simulink model "demoProxyRPi"  (R2016a)
settings: Solver=FixedStepAuto  StartTime=0.0  StopTime=inf  FixedStep=1  RelTol=1e-3
undefined symbols (not defined in the file): Green, led0
libraries: embdlinuxlib x3, RPi x2
settings Model: SimulationMode=external  Creator=user  LastModifiedBy=user
settings SolverCC: PositivePriorityOrder=on
settings OptimizationCC: OptimizeModelRefInitCode=on  LifeSpan=1  MaxStackSize=64
settings HardwareCC: ProdBitPerPointer=32  ProdLargestAtomicInteger=Long  ProdLargestAtomicFloat=Double  ProdWordSize=32  ProdHWDeviceType=ARM Compatible->ARM Cortex
settings RTWCC: SystemTargetFile=ert.tlc  HardwareBoard=Raspberry Pi  TemplateMakefile=ert_default_tmf  GenerateReport=on  Toolchain=GNU GCC Raspberry Pi  IncludeHyperlinkInReport=on  LaunchReport=on  GenerateTraceInfo=on  GenerateTraceReport=on  GenerateTraceReportSl=on  GenerateTraceReportSf=on  GenerateTraceReportEml=on
settings CodeAppCC: ForceParamTrailComments=on  IgnoreCustomStorageClasses=off  OperatorAnnotations=on  SimulinkDataObjDesc=on  SFDataObjDesc=on  MATLABFcnDesc=on  InsertBlockDesc=on  MATLABSourceComments=on
settings ERTTargetCC: SupportVariableSizeSignals=on

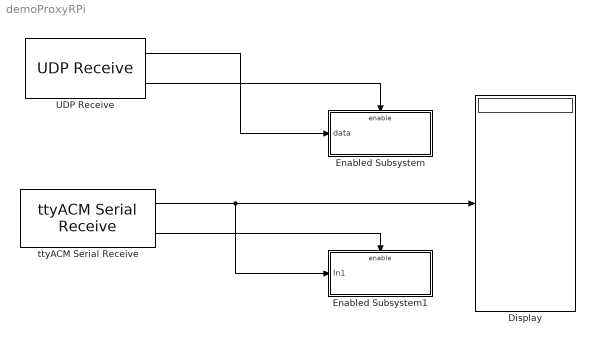
== system demoProxyRPi ==
  Display : Display
  Enabled Subsystem : Subsystem  TreatAsAtomicUnit=on
  Enabled Subsystem1 : Subsystem  TreatAsAtomicUnit=on
  UDP Receive : embdlinuxlib/UDP Receive  localURL='0.0.0.0'  localPort=25000  remoteURL='0.0.0.0'  remotePort=-1  recvBufferSize=8192  signalDatatype=uint8  dims=10  isVarSize=off  showBlockingTime=off  blockingTime=0  sampletime=1  blockPlatform=Raspberry Pi
  ttyACM Serial Receive : RPi/ttyACM Serial Receive  portID=0  msgLen=10  SimulateUsing=Code generation
  wires:
  UDP Receive/2 -> Enabled Subsystem/Enable
  UDP Receive/1 -> Enabled Subsystem/1(data)
  ttyACM Serial Receive/2 -> Enabled Subsystem1/Enable
  ttyACM Serial Receive/1 -> Enabled Subsystem1/1(In1), Display/1

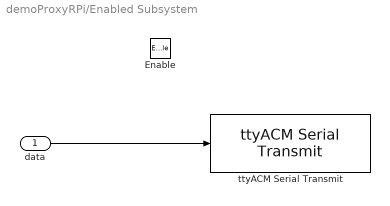
== system demoProxyRPi/Enabled Subsystem ==
  data : Inport
  Enable : EnablePort
  ttyACM Serial Transmit : RPi/ttyACM Serial Transmit  portID=0  SimulateUsing=Code generation
  wires:
  data/1 -> ttyACM Serial Transmit/1

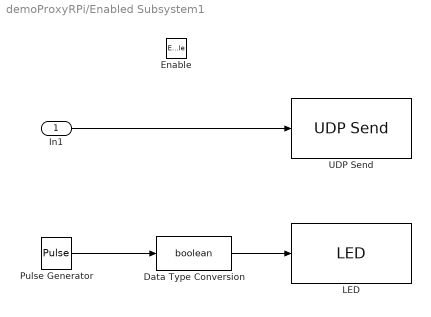
== system demoProxyRPi/Enabled Subsystem1 ==
  In1 : Inport
  Enable : EnablePort
  Data Type Conversion : DataTypeConversion  OutDataTypeStr=boolean
  LED : embdlinuxlib/LED  board=Pi 3 Model B  led=led0 (Green)  blockPlatform=Raspberry Pi
  Pulse Generator : DiscretePulseGenerator  SampleTime=-1
  UDP Send : embdlinuxlib/UDP Send  remoteURL='255.255.255.255'  remotePort=25001  localURL='255.255.255.255'  localPortSource=Automatically determine  localPort=-1  sampletime=-1  blockPlatform=Raspberry Pi  separateLengthPort=0
  wires:
  In1/1 -> UDP Send/1
  Data Type Conversion/1 -> LED/1
  Pulse Generator/1 -> Data Type Conversion/1
